simulink model "myFirstSystemModel"  (R2022a)
settings: Solver=VariableStepAuto  StartTime=0.0  StopTime=10.0  RelTol=1e-3
settings Model: Creator=mrnel  LastModifiedBy=mrnel

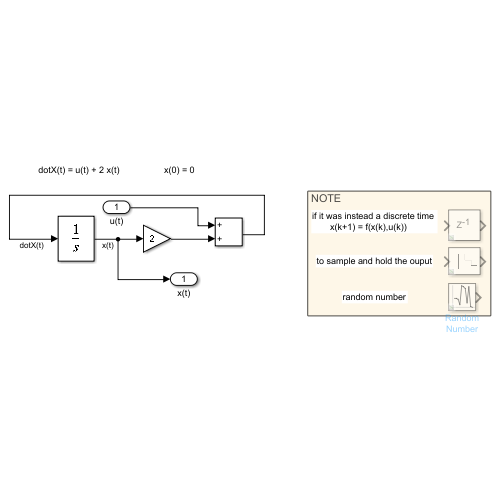
[thumbnail: Simulink's stored preview of the top-level diagram]
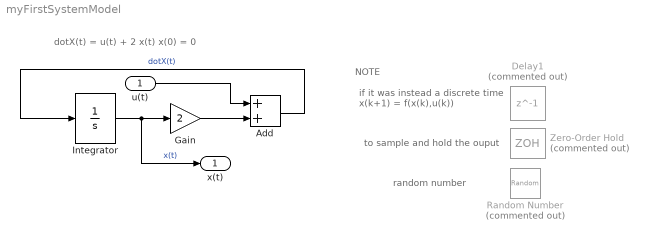
== system myFirstSystemModel ==
  note: NOTE
  note: dotX(t) = u(t) + 2 x(t) x(0) = 0
  note: if it was instead a discrete time
      | 	x(k+1) = f(x(k),u(k))
  note: to sample and hold the ouput
  note: random number
  u(t) : Inport
  Add : Sum
  Delay1 : Delay  Commented=on  DelayLength=1  InitialCondition=0
  Gain : Gain  Gain=2
  Integrator : Integrator
  Random Number : RandomNumber  Commented=on  SampleTime=0.1
  Zero-Order Hold : ZeroOrderHold  Commented=on  SampleTime=-1
  x(t) : Outport
  wires:
  Integrator/1 -> x(t)/1, Gain/1  "x(t)"
  u(t)/1 -> Add/1
  Add/1 -> Integrator/1  "dotX(t)"
  Gain/1 -> Add/2
